simulink model "XGGDZhPID"  (Simulink 5.0)
settings: Solver=ode4  StartTime=0.0  StopTime=8000  FixedStep=20  RelTol=1e-3
settings Model: LastModifiedBy=ThinkPad

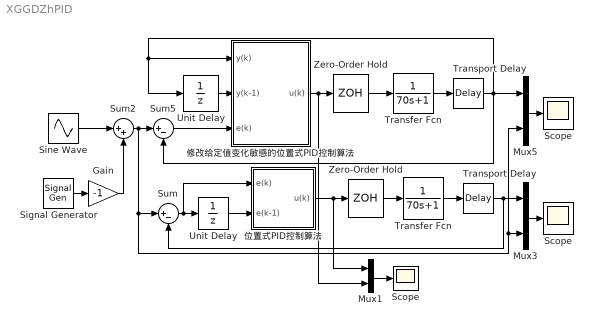
== system XGGDZhPID ==
  " Scope " : Scope
      settings: YMin=-1.3  YMax=1.3  SaveName=PID  DataFormat=Array  MaxDataPoints=500000
  " 修改给定值变化敏感的位置式PID控制算法" : Subsystem
  Gain : Gain  Gain=-1  SaturateOnIntegerOverflow=on
  Mux1 : Mux  Inputs=2
  Mux3 : Mux  Inputs=2
  Mux5 : Mux  Inputs=2
  Scope : Scope
      settings: YMin=-1.3  YMax=1.3  SaveName=XGGDZhPIDry  DataFormat=Array  MaxDataPoints=500000
  "Scope " : Scope
      settings: YMin=-1.5  YMax=1.5  SaveName=XGGDZhPIDu  DataFormat=Array  MaxDataPoints=500000
  Signal Generator : SignalGenerator  WaveForm=square  Frequency=0.0005*pi  Units=rad/sec
  Sine Wave : Sin  Amplitude=0.05  Frequency=0.03*pi  SampleTime=0
  Sum : Sum  Inputs=|+-  SaturateOnIntegerOverflow=on
  Sum2 : Sum  Inputs=|++  SaturateOnIntegerOverflow=on
  Sum5 : Sum  Inputs=|+-  SaturateOnIntegerOverflow=on
  Transfer Fcn : TransferFcn  Denominator=[70 1]
  "Transfer Fcn " : TransferFcn  Denominator=[70 1]
  Transport Delay : TransportDelay  DelayTime=80
  "Transport Delay " : TransportDelay  DelayTime=80
  Unit Delay : UnitDelay  SampleTime=20
  "Unit Delay " : UnitDelay  SampleTime=20
  Zero-Order Hold : ZeroOrderHold  SampleTime=20
  "Zero-Order Hold " : ZeroOrderHold  SampleTime=20
  "位置式PID控制算法 " : Subsystem
  wires:
  Sine Wave/1 -> Sum2/1
  Signal Generator/1 -> Gain/1
  Gain/1 -> Sum2/2
  Sum2/1 -> Sum5/1, Sum/1, Mux5/2, Mux3/2
  Transfer Fcn/1 -> Transport Delay/1
  Zero-Order Hold/1 -> Transfer Fcn/1
  Mux5/1 -> Scope/1
  Transport Delay/1 -> Mux5/1, Sum5/2, "Unit Delay "/1, " 修改给定值变化敏感的位置式PID控制算法"/1(y(k))
  " 修改给定值变化敏感的位置式PID控制算法"/1(u(k)) -> Zero-Order Hold/1, Mux1/2
  Sum5/1 -> " 修改给定值变化敏感的位置式PID控制算法"/3(e(k))
  "Unit Delay "/1 -> " 修改给定值变化敏感的位置式PID控制算法"/2(y(k-1))
  Sum/1 -> "位置式PID控制算法 "/1(e(k)), Unit Delay/1
  "位置式PID控制算法 "/1(u(k)) -> "Zero-Order Hold "/1, Mux1/1
  Mux3/1 -> " Scope "/1
  "Transfer Fcn "/1 -> "Transport Delay "/1
  "Zero-Order Hold "/1 -> "Transfer Fcn "/1
  "Transport Delay "/1 -> Sum/2, Mux3/1
  Unit Delay/1 -> "位置式PID控制算法 "/2(e(k-1))
  Mux1/1 -> "Scope "/1

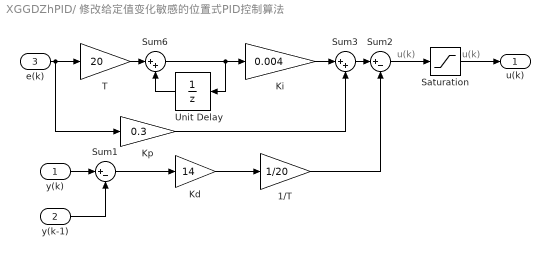
== system XGGDZhPID/ 修改给定值变化敏感的位置式PID控制算法 ==
  note: u(k)
  note: u(k)
  y(k) : Inport
  y(k-1) : Inport  Port=2
  e(k) : Inport  Port=3
  1/T : Gain  Gain=1/20  SaturateOnIntegerOverflow=on
  Kd : Gain  Gain=14  SaturateOnIntegerOverflow=on
  Ki : Gain  Gain=0.004  SaturateOnIntegerOverflow=on
  Kp : Gain  Gain=0.3  SaturateOnIntegerOverflow=on
  Saturation : Saturate  UpperLimit=10  LowerLimit=-10
  Sum1 : Sum  Inputs=|+-  SaturateOnIntegerOverflow=on
  Sum2 : Sum  Inputs=|+-  SaturateOnIntegerOverflow=on
  Sum3 : Sum  Inputs=|++  SaturateOnIntegerOverflow=on
  Sum6 : Sum  Inputs=|++  SaturateOnIntegerOverflow=on
  T : Gain  Gain=20  SaturateOnIntegerOverflow=on
  "Unit Delay " : UnitDelay  Orientation=left  SampleTime=20
  u(k) : Outport
  wires:
  e(k)/1 -> T/1, Kp/1
  y(k-1)/1 -> Sum1/2
  y(k)/1 -> Sum1/1
  Sum1/1 -> Kd/1
  Kd/1 -> 1/T/1
  Saturation/1 -> u(k)/1
  Kp/1 -> Sum3/2
  Ki/1 -> Sum3/1
  T/1 -> Sum6/1
  "Unit Delay "/1 -> Sum6/2
  Sum6/1 -> "Unit Delay "/1, Ki/1
  Sum3/1 -> Sum2/1
  Sum2/1 -> Saturation/1
  1/T/1 -> Sum2/2

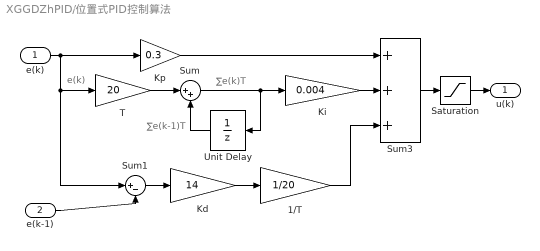
== system XGGDZhPID/位置式PID控制算法  ==
  note: e(k)
  note: ∑e(k)T
  note: ∑e(k-1)T
  e(k) : Inport
  e(k-1) : Inport  Port=2
  1/T : Gain  Gain=1/20  SaturateOnIntegerOverflow=on
  Kd : Gain  Gain=14  SaturateOnIntegerOverflow=on
  Ki : Gain  Gain=0.004  SaturateOnIntegerOverflow=on
  Kp : Gain  Gain=0.3  SaturateOnIntegerOverflow=on
  Saturation : Saturate  UpperLimit=10  LowerLimit=-10
  Sum : Sum  Inputs=|++  SaturateOnIntegerOverflow=on
  Sum1 : Sum  Inputs=|+-  SaturateOnIntegerOverflow=on
  Sum3 : Sum  Inputs=+++  SaturateOnIntegerOverflow=on
  T : Gain  Gain=20  SaturateOnIntegerOverflow=on
  Unit Delay : UnitDelay  Orientation=left  SampleTime=20
  u(k) : Outport
  wires:
  Sum1/1 -> Kd/1
  e(k)/1 -> Kp/1, Sum1/1, T/1
  Kp/1 -> Sum3/1
  Ki/1 -> Sum3/2
  Sum3/1 -> Saturation/1
  Kd/1 -> 1/T/1
  1/T/1 -> Sum3/3
  Sum/1 -> Unit Delay/1, Ki/1
  Unit Delay/1 -> Sum/2
  e(k-1)/1 -> Sum1/2
  T/1 -> Sum/1
  Saturation/1 -> u(k)/1
